simulink subsystem "AngVelocitySignals"  (R2021a)
settings: Solver=VariableStepAuto  StartTime=0.0  StopTime=10.0  RelTol=1e-3
undefined symbols (not defined in the file): t0x, t0y, t0z, tfx, tfy, tfz, wx, wy, wz
settings Model: Creator=Laura  LastModifiedBy=Laura

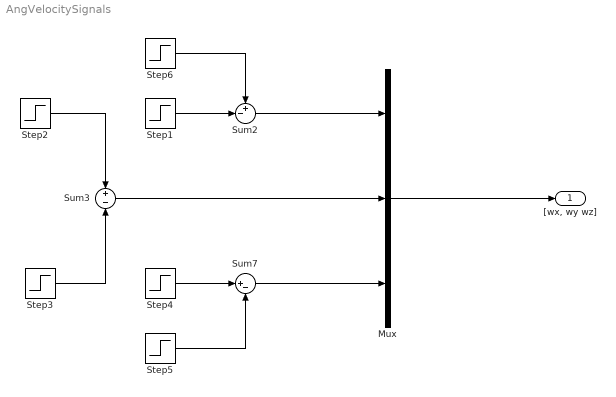
== system AngVelocitySignals ==
  Mux : Mux  Inputs=3
  Step1 : Step  Time=tfx  After=wx  SampleTime=0
  Step2 : Step  Time=t0y  After=wy  SampleTime=0
  Step3 : Step  Time=tfy  After=wy  SampleTime=0
  Step4 : Step  Time=t0z  After=wz  SampleTime=0
  Step5 : Step  Time=tfz  After=wz  SampleTime=0
  Step6 : Step  Time=t0x  After=wx  SampleTime=0
  Sum2 : Sum  Inputs=+-|
  Sum3 : Sum  Inputs=+-
  Sum7 : Sum  Inputs=|+-
  "[wx, wy wz]" : Outport
  wires:
  Step6/1 -> Sum2/1
  Sum3/1 -> Mux/2
  Sum7/1 -> Mux/3
  Mux/1 -> "[wx, wy wz]"/1
  Step1/1 -> Sum2/2
  Step4/1 -> Sum7/1
  Step3/1 -> Sum3/2
  Sum2/1 -> Mux/1
  Step5/1 -> Sum7/2
  Step2/1 -> Sum3/1
